simulink model "Controllers_Disturbances"  (R2019a)
settings: Solver=VariableStepAuto  StartTime=0.0  StopTime=50  RelTol=1e-3
PreLoadFcn:
  | Setup_VariantControl
undefined symbols (not defined in the file or in its folder): controller_H2, controller_INF, controller_LQR, plant_aug
settings Model: Creator=martin  LastModifiedBy=martin

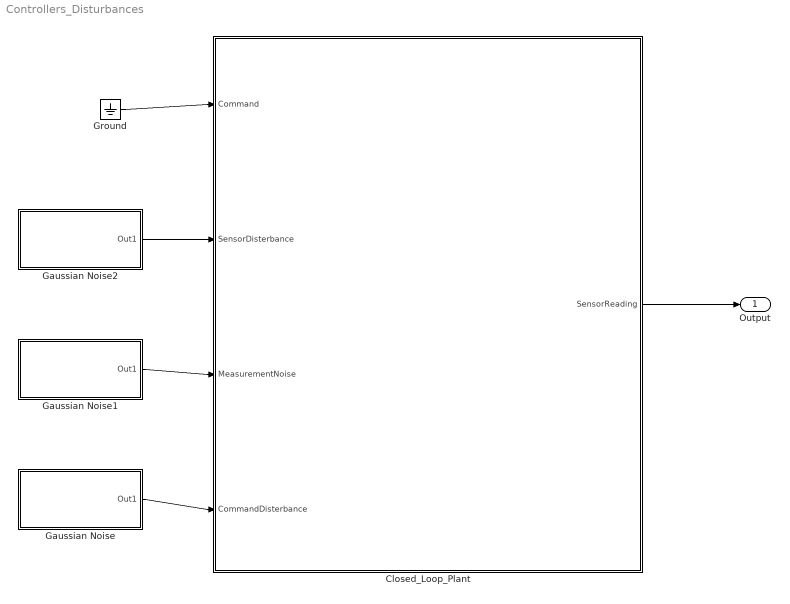
== system Controllers_Disturbances ==
  Closed_Loop_Plant : Subsystem  Variant=on  VariantControl=Variant1
  Gaussian Noise : Subsystem
  Gaussian Noise1 : Subsystem
  Gaussian Noise2 : Subsystem
  Ground : Ground
  Output : Outport
  wires:
  Gaussian Noise/1(Out1) -> Closed_Loop_Plant/4(CommandDisterbance)
  Gaussian Noise1/1(Out1) -> Closed_Loop_Plant/3(MeasurementNoise)
  Gaussian Noise2/1(Out1) -> Closed_Loop_Plant/2(SensorDisterbance)
  Ground/1 -> Closed_Loop_Plant/1(Command)
  Closed_Loop_Plant/1(SensorReading) -> Output/1

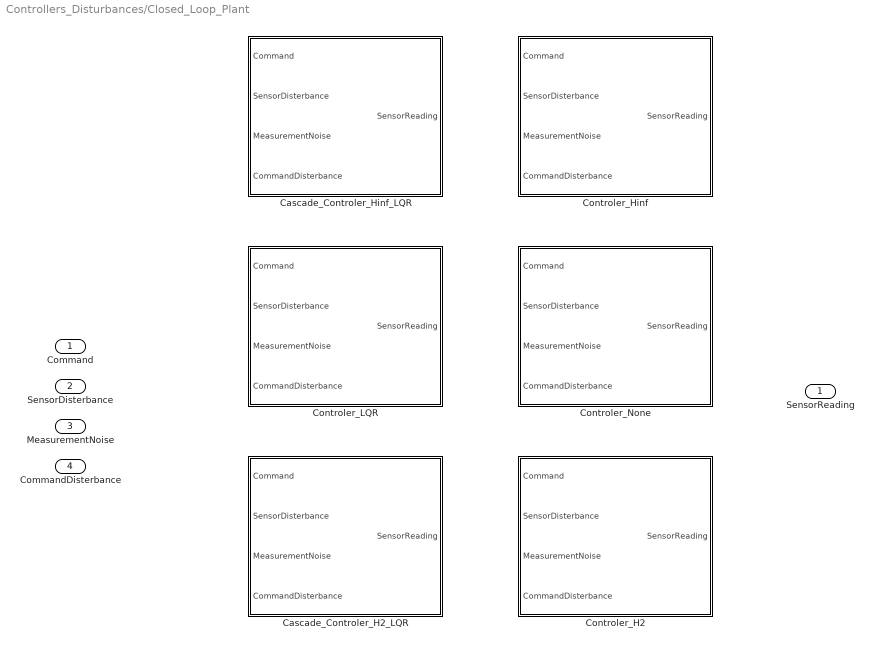
== system Controllers_Disturbances/Closed_Loop_Plant ==
  Command : Inport
  SensorDisterbance : Inport  Port=2
  MeasurementNoise : Inport  Port=3
  CommandDisterbance : Inport  Port=4
  Cascade_Controler_H2_LQR : Subsystem  VariantControl=VC_H2_LQR
  Cascade_Controler_Hinf_LQR : Subsystem  VariantControl=VC_Cascade_Hinf_LQR
  Controler_H2 : Subsystem  VariantControl=VC_H2
  Controler_Hinf : Subsystem  VariantControl=VC_Hinf
  Controler_LQR : Subsystem  VariantControl=VC_LQR
  Controler_None : Subsystem  VariantControl=VC_None
  SensorReading : Outport

== system Controllers_Disturbances/Gaussian Noise ==
  Gausian Noise : MATLAB Function  TreatAsAtomicUnit=on
  Ground : Ground
  Variant Source : VariantSource
  Out1 : Outport
  wires:
  Ground/1 -> Variant Source/2  "No_noise"
  Gausian Noise/1(noise) -> Variant Source/1
  Variant Source/1 -> Out1/1

== system Controllers_Disturbances/Gaussian Noise1 ==
  Gausian Noise : MATLAB Function  TreatAsAtomicUnit=on
  Ground : Ground
  Variant Source : VariantSource
  Out1 : Outport
  wires:
  Variant Source/1 -> Out1/1
  Gausian Noise/1(noise) -> Variant Source/1
  Ground/1 -> Variant Source/2  "No_noise"

== system Controllers_Disturbances/Gaussian Noise2 ==
  Gausian Noise : MATLAB Function  TreatAsAtomicUnit=on
  Ground : Ground
  Variant Source : VariantSource
  Out1 : Outport
  wires:
  Ground/1 -> Variant Source/2  "No_noise"
  Gausian Noise/1(noise) -> Variant Source/1
  Variant Source/1 -> Out1/1

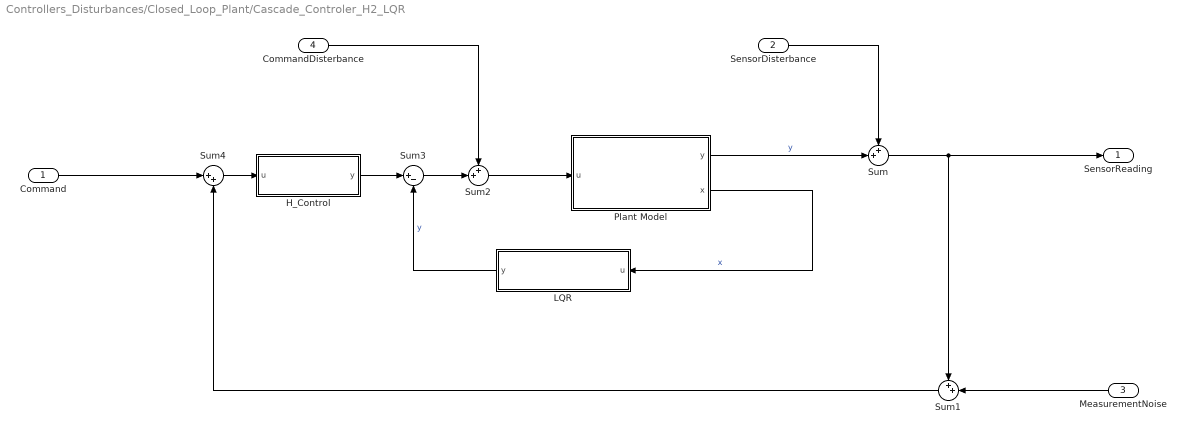
== system Controllers_Disturbances/Closed_Loop_Plant/Cascade_Controler_H2_LQR ==
  Command : Inport
  SensorDisterbance : Inport  Port=2  PortDimensions=1
  MeasurementNoise : Inport  Port=3  PortDimensions=1
  CommandDisterbance : Inport  Port=4  PortDimensions=1
  H_Control : Subsystem  mask{plant=controller_H2, IC=[0,0,0,0]'}
      mask prompts: plant "Plant SS Object"; IC "Inital Conditions"
  LQR : Subsystem  mask{plant=controller_LQR, IC=[0]'}
      mask prompts: plant "Plant SS Object"; IC "Inital Conditions"
  Plant Model : Subsystem  mask{plant=plant_aug, IC=[0,0]'}
      mask prompts: plant "Plant SS Object"; IC "Inital Conditions"
  Sum : Sum  Inputs=++|
  Sum1 : Sum  Inputs=++|
  Sum2 : Sum  Inputs=++|
  Sum3 : Sum  Inputs=|+-
  Sum4 : Sum  Inputs=|++
  SensorReading : Outport  PortDimensions=1
  wires:
  Sum4/1 -> H_Control/1(u)
  H_Control/1(y) -> Sum3/1
  Sum1/1 -> Sum4/2
  LQR/1(y) -> Sum3/2  "y"
  Plant Model/2(x) -> LQR/1(u)  "x"
  MeasurementNoise/1 -> Sum1/2
  Plant Model/1(y) -> Sum/2  "y"
  Sum2/1 -> Plant Model/1(u)
  Command/1 -> Sum4/1
  CommandDisterbance/1 -> Sum2/1
  Sum3/1 -> Sum2/2
  Sum/1 -> Sum1/1, SensorReading/1
  SensorDisterbance/1 -> Sum/1

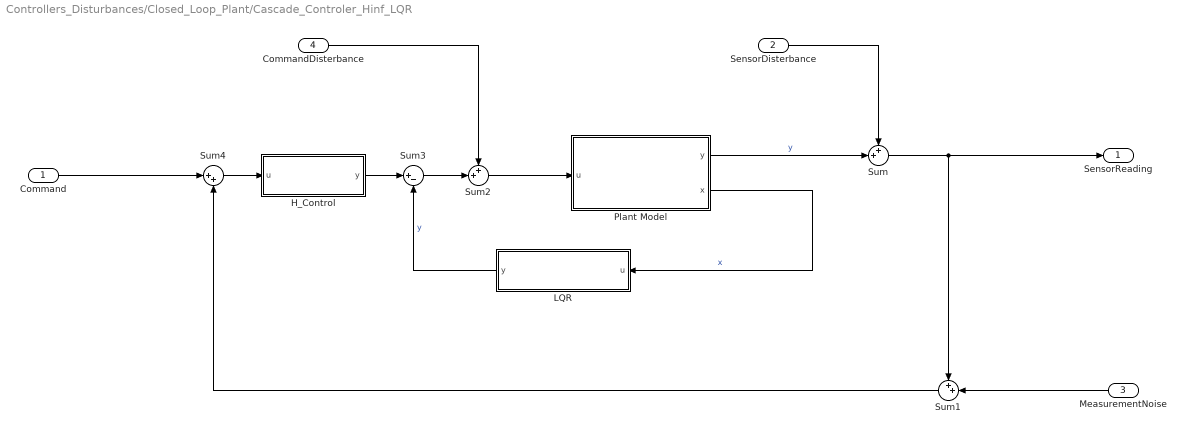
== system Controllers_Disturbances/Closed_Loop_Plant/Cascade_Controler_Hinf_LQR ==
  Command : Inport
  SensorDisterbance : Inport  Port=2  PortDimensions=1
  MeasurementNoise : Inport  Port=3  PortDimensions=1
  CommandDisterbance : Inport  Port=4  PortDimensions=1
  H_Control : Subsystem  mask{plant=controller_INF, IC=[0,0,0,0]'}
      mask prompts: plant "Plant SS Object"; IC "Inital Conditions"
  LQR : Subsystem  mask{plant=controller_LQR, IC=[0]'}
      mask prompts: plant "Plant SS Object"; IC "Inital Conditions"
  Plant Model : Subsystem  mask{plant=plant_aug, IC=[0,0]'}
      mask prompts: plant "Plant SS Object"; IC "Inital Conditions"
  Sum : Sum  Inputs=++|
  Sum1 : Sum  Inputs=++|
  Sum2 : Sum  Inputs=++|
  Sum3 : Sum  Inputs=|+-
  Sum4 : Sum  Inputs=|++
  SensorReading : Outport  PortDimensions=1
  wires:
  SensorDisterbance/1 -> Sum/1
  Sum/1 -> SensorReading/1, Sum1/1
  Sum3/1 -> Sum2/2
  CommandDisterbance/1 -> Sum2/1
  Command/1 -> Sum4/1
  Sum2/1 -> Plant Model/1(u)
  Plant Model/1(y) -> Sum/2  "y"
  MeasurementNoise/1 -> Sum1/2
  Plant Model/2(x) -> LQR/1(u)  "x"
  LQR/1(y) -> Sum3/2  "y"
  Sum1/1 -> Sum4/2
  H_Control/1(y) -> Sum3/1
  Sum4/1 -> H_Control/1(u)

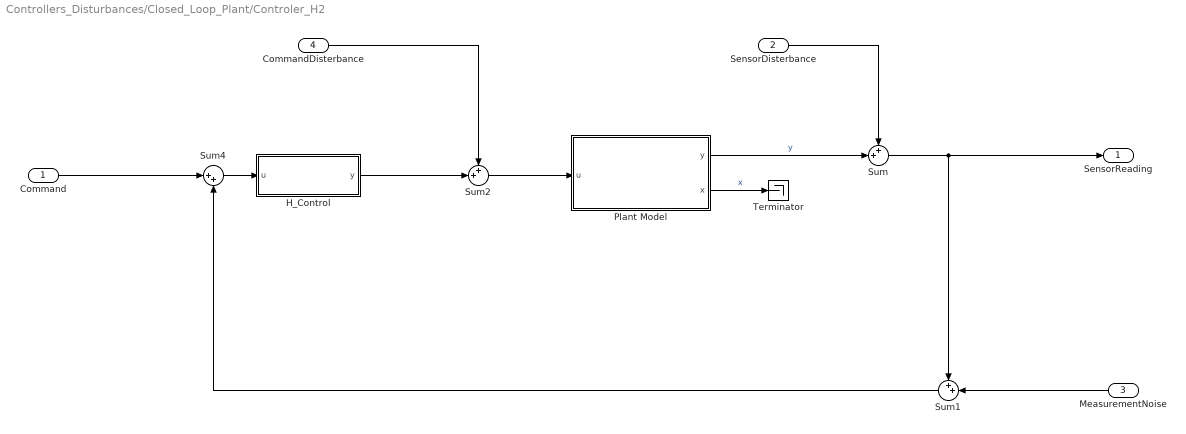
== system Controllers_Disturbances/Closed_Loop_Plant/Controler_H2 ==
  Command : Inport
  SensorDisterbance : Inport  Port=2  PortDimensions=1
  MeasurementNoise : Inport  Port=3  PortDimensions=1
  CommandDisterbance : Inport  Port=4  PortDimensions=1
  H_Control : Subsystem  mask{plant=controller_H2, IC=[0,0,0,0]'}
      mask prompts: plant "Plant SS Object"; IC "Inital Conditions"
  Plant Model : Subsystem  mask{plant=plant_aug, IC=[0,0]'}
      mask prompts: plant "Plant SS Object"; IC "Inital Conditions"
  Sum : Sum  Inputs=++|
  Sum1 : Sum  Inputs=++|
  Sum2 : Sum  Inputs=++|
  Sum4 : Sum  Inputs=|++
  Terminator : Terminator
  SensorReading : Outport  PortDimensions=1
  wires:
  SensorDisterbance/1 -> Sum/1
  Sum/1 -> SensorReading/1, Sum1/1
  H_Control/1(y) -> Sum2/2
  CommandDisterbance/1 -> Sum2/1
  Command/1 -> Sum4/1
  Sum2/1 -> Plant Model/1(u)
  Plant Model/1(y) -> Sum/2  "y"
  MeasurementNoise/1 -> Sum1/2
  Plant Model/2(x) -> Terminator/1  "x"
  Sum1/1 -> Sum4/2
  Sum4/1 -> H_Control/1(u)

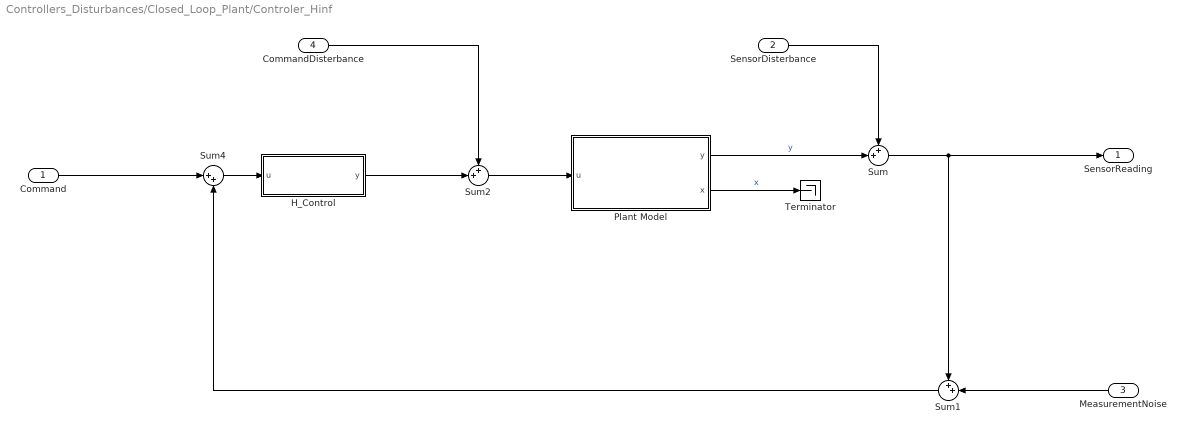
== system Controllers_Disturbances/Closed_Loop_Plant/Controler_Hinf ==
  Command : Inport
  SensorDisterbance : Inport  Port=2  PortDimensions=1
  MeasurementNoise : Inport  Port=3  PortDimensions=1
  CommandDisterbance : Inport  Port=4  PortDimensions=1
  H_Control : Subsystem  mask{plant=controller_INF, IC=[0,0,0,0]'}
      mask prompts: plant "Plant SS Object"; IC "Inital Conditions"
  Plant Model : Subsystem  mask{plant=plant_aug, IC=[0,0]'}
      mask prompts: plant "Plant SS Object"; IC "Inital Conditions"
  Sum : Sum  Inputs=++|
  Sum1 : Sum  Inputs=++|
  Sum2 : Sum  Inputs=++|
  Sum4 : Sum  Inputs=|++
  Terminator : Terminator
  SensorReading : Outport  PortDimensions=1
  wires:
  Sum4/1 -> H_Control/1(u)
  Sum1/1 -> Sum4/2
  Plant Model/2(x) -> Terminator/1  "x"
  MeasurementNoise/1 -> Sum1/2
  Plant Model/1(y) -> Sum/2  "y"
  Sum2/1 -> Plant Model/1(u)
  Command/1 -> Sum4/1
  CommandDisterbance/1 -> Sum2/1
  H_Control/1(y) -> Sum2/2
  Sum/1 -> Sum1/1, SensorReading/1
  SensorDisterbance/1 -> Sum/1

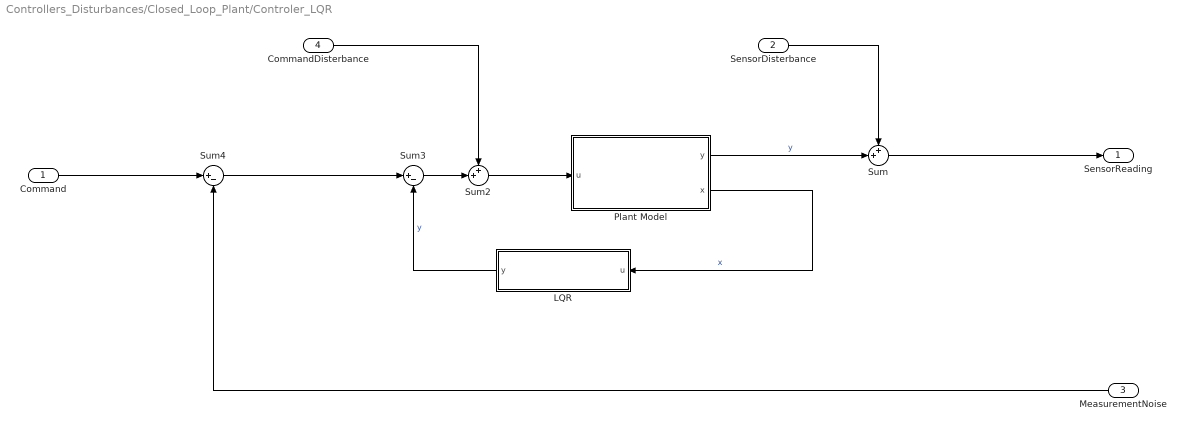
== system Controllers_Disturbances/Closed_Loop_Plant/Controler_LQR ==
  Command : Inport
  SensorDisterbance : Inport  Port=2  PortDimensions=1
  MeasurementNoise : Inport  Port=3  PortDimensions=1
  CommandDisterbance : Inport  Port=4  PortDimensions=1
  LQR : Subsystem  mask{plant=controller_LQR, IC=[0]'}
      mask prompts: plant "Plant SS Object"; IC "Inital Conditions"
  Plant Model : Subsystem  mask{plant=plant_aug, IC=[0,0]'}
      mask prompts: plant "Plant SS Object"; IC "Inital Conditions"
  Sum : Sum  Inputs=++|
  Sum2 : Sum  Inputs=++|
  Sum3 : Sum  Inputs=|+-
  Sum4 : Sum  Inputs=|+-
  SensorReading : Outport  PortDimensions=1
  wires:
  Sum4/1 -> Sum3/1
  MeasurementNoise/1 -> Sum4/2
  LQR/1(y) -> Sum3/2  "y"
  Plant Model/2(x) -> LQR/1(u)  "x"
  Plant Model/1(y) -> Sum/2  "y"
  Sum2/1 -> Plant Model/1(u)
  Command/1 -> Sum4/1
  CommandDisterbance/1 -> Sum2/1
  Sum3/1 -> Sum2/2
  Sum/1 -> SensorReading/1
  SensorDisterbance/1 -> Sum/1

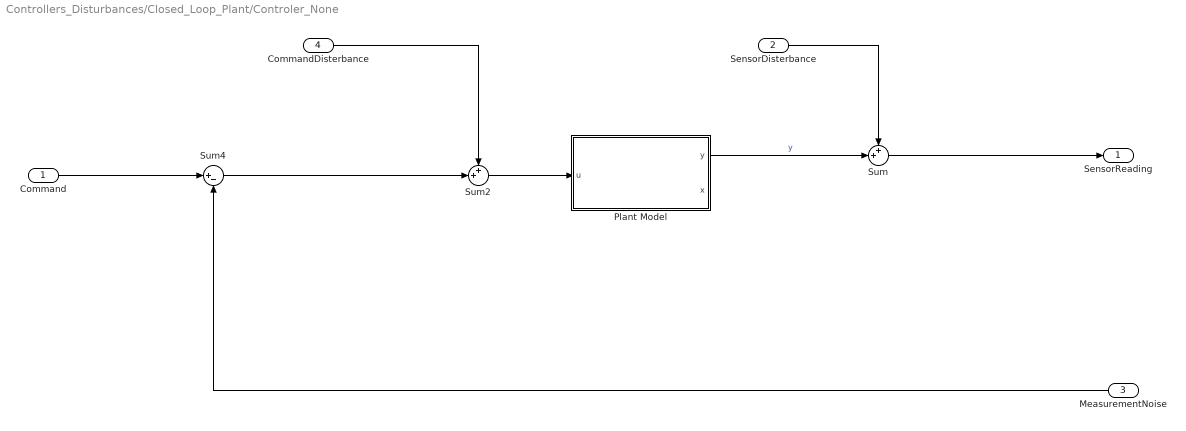
== system Controllers_Disturbances/Closed_Loop_Plant/Controler_None ==
  Command : Inport
  SensorDisterbance : Inport  Port=2  PortDimensions=1
  MeasurementNoise : Inport  Port=3  PortDimensions=1
  CommandDisterbance : Inport  Port=4  PortDimensions=1
  Plant Model : Subsystem  mask{plant=plant_aug, IC=[0,0]'}
      mask prompts: plant "Plant SS Object"; IC "Inital Conditions"
  Sum : Sum  Inputs=++|
  Sum2 : Sum  Inputs=++|
  Sum4 : Sum  Inputs=|+-
  SensorReading : Outport  PortDimensions=1
  wires:
  SensorDisterbance/1 -> Sum/1
  Sum/1 -> SensorReading/1
  Sum4/1 -> Sum2/2
  CommandDisterbance/1 -> Sum2/1
  Command/1 -> Sum4/1
  Sum2/1 -> Plant Model/1(u)
  Plant Model/1(y) -> Sum/2  "y"
  MeasurementNoise/1 -> Sum4/2

== system Controllers_Disturbances/Closed_Loop_Plant/Cascade_Controler_H2_LQR/H_Control ==
  u : Inport
  State-Space : StateSpace  A=plant.A  B=plant.B  C=plant.C  D=plant.D  InitialCondition=IC
  y : Outport
  wires:
  State-Space/1 -> y/1
  u/1 -> State-Space/1

== system Controllers_Disturbances/Closed_Loop_Plant/Cascade_Controler_H2_LQR/LQR ==
  u : Inport
  State-Space : StateSpace  A=plant.A  B=plant.B  C=plant.C  D=plant.D  InitialCondition=IC
  y : Outport
  wires:
  u/1 -> State-Space/1
  State-Space/1 -> y/1

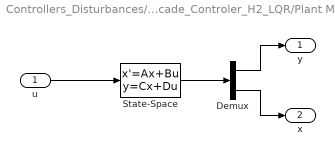
== system Controllers_Disturbances/Closed_Loop_Plant/Cascade_Controler_H2_LQR/Plant Model ==
  u : Inport
  Demux : Demux  Outputs=[1,2]
  State-Space : StateSpace  A=plant.A  B=plant.B  C=plant.C  D=plant.D  InitialCondition=IC
  y : Outport
  x : Outport  Port=2
  wires:
  Demux/2 -> x/1
  Demux/1 -> y/1
  u/1 -> State-Space/1
  State-Space/1 -> Demux/1

== system Controllers_Disturbances/Closed_Loop_Plant/Cascade_Controler_Hinf_LQR/H_Control ==
  u : Inport
  State-Space : StateSpace  A=plant.A  B=plant.B  C=plant.C  D=plant.D  InitialCondition=IC
  y : Outport
  wires:
  u/1 -> State-Space/1
  State-Space/1 -> y/1

== system Controllers_Disturbances/Closed_Loop_Plant/Cascade_Controler_Hinf_LQR/LQR ==
  u : Inport
  State-Space : StateSpace  A=plant.A  B=plant.B  C=plant.C  D=plant.D  InitialCondition=IC
  y : Outport
  wires:
  State-Space/1 -> y/1
  u/1 -> State-Space/1

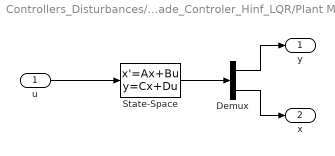
== system Controllers_Disturbances/Closed_Loop_Plant/Cascade_Controler_Hinf_LQR/Plant Model ==
  u : Inport
  Demux : Demux  Outputs=[1,2]
  State-Space : StateSpace  A=plant.A  B=plant.B  C=plant.C  D=plant.D  InitialCondition=IC
  y : Outport
  x : Outport  Port=2
  wires:
  State-Space/1 -> Demux/1
  u/1 -> State-Space/1
  Demux/1 -> y/1
  Demux/2 -> x/1

== system Controllers_Disturbances/Closed_Loop_Plant/Controler_H2/H_Control ==
  u : Inport
  State-Space : StateSpace  A=plant.A  B=plant.B  C=plant.C  D=plant.D  InitialCondition=IC
  y : Outport
  wires:
  u/1 -> State-Space/1
  State-Space/1 -> y/1

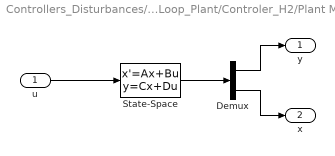
== system Controllers_Disturbances/Closed_Loop_Plant/Controler_H2/Plant Model ==
  u : Inport
  Demux : Demux  Outputs=[1,2]
  State-Space : StateSpace  A=plant.A  B=plant.B  C=plant.C  D=plant.D  InitialCondition=IC
  y : Outport
  x : Outport  Port=2
  wires:
  State-Space/1 -> Demux/1
  u/1 -> State-Space/1
  Demux/1 -> y/1
  Demux/2 -> x/1

== system Controllers_Disturbances/Closed_Loop_Plant/Controler_Hinf/H_Control ==
  u : Inport
  State-Space : StateSpace  A=plant.A  B=plant.B  C=plant.C  D=plant.D  InitialCondition=IC
  y : Outport
  wires:
  State-Space/1 -> y/1
  u/1 -> State-Space/1

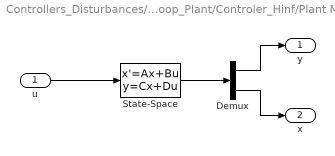
== system Controllers_Disturbances/Closed_Loop_Plant/Controler_Hinf/Plant Model ==
  u : Inport
  Demux : Demux  Outputs=[1,2]
  State-Space : StateSpace  A=plant.A  B=plant.B  C=plant.C  D=plant.D  InitialCondition=IC
  y : Outport
  x : Outport  Port=2
  wires:
  Demux/2 -> x/1
  Demux/1 -> y/1
  u/1 -> State-Space/1
  State-Space/1 -> Demux/1

== system Controllers_Disturbances/Closed_Loop_Plant/Controler_LQR/LQR ==
  u : Inport
  State-Space : StateSpace  A=plant.A  B=plant.B  C=plant.C  D=plant.D  InitialCondition=IC
  y : Outport
  wires:
  u/1 -> State-Space/1
  State-Space/1 -> y/1

== system Controllers_Disturbances/Closed_Loop_Plant/Controler_LQR/Plant Model ==
  u : Inport
  Demux : Demux  Outputs=[1,2]
  State-Space : StateSpace  A=plant.A  B=plant.B  C=plant.C  D=plant.D  InitialCondition=IC
  y : Outport
  x : Outport  Port=2
  wires:
  Demux/2 -> x/1
  Demux/1 -> y/1
  u/1 -> State-Space/1
  State-Space/1 -> Demux/1

== system Controllers_Disturbances/Closed_Loop_Plant/Controler_None/Plant Model ==
  u : Inport
  Demux : Demux  Outputs=[1,2]
  State-Space : StateSpace  A=plant.A  B=plant.B  C=plant.C  D=plant.D  InitialCondition=IC
  y : Outport
  x : Outport  Port=2
  wires:
  State-Space/1 -> Demux/1
  u/1 -> State-Space/1
  Demux/1 -> y/1
  Demux/2 -> x/1

== matlab function Controllers_Disturbances/Gaussian Noise1/Gausian Noise ==
  data: noise output; power parameter
function noise = fcn(power)
noise = wgn(1,1,power);

== matlab function Controllers_Disturbances/Gaussian Noise/Gausian Noise ==
  data: noise output; power parameter
function noise = fcn(power)
noise = wgn(1,1,power);

== matlab function Controllers_Disturbances/Gaussian Noise2/Gausian Noise ==
  data: noise output; power parameter
function noise = fcn(power)
noise = wgn(1,1,power);
